simulink model "BSCU"  (R2014b)
settings: Solver=ode45  StartTime=0.0  StopTime=10.0  RelTol=1e-3
undefined symbols (not defined in the file): BRAKE_PRESSURE_LO, BRAKE_PRESSURE_MAX, BRAKE_PRESSURE_MED, LO, MANUAL, MAX, MED
settings Model: CovSFcnEnable=on  Creator=hamza  LastModifiedBy=hbourbou
settings DataIOCC: LimitDataPoints=off  SaveFormat=StructureWithTime
settings DebuggingCC: SolverPrmCheckMsg=none  FrameProcessingCompatibilityMsg=error
settings HardwareCC: ProdBitPerPointer=64  ProdLargestAtomicFloat=Float  ProdIntDivRoundTo=Zero  ProdEndianess=LittleEndian  ProdHWDeviceType=Specified
settings ModelReferenceCC: PropagateSignalLabelsOutOfModel=on

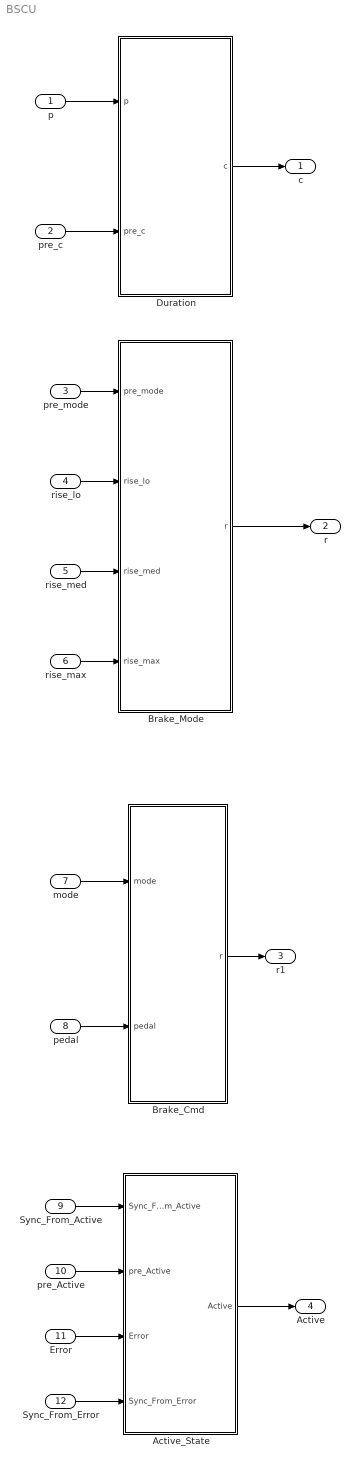
== system BSCU ==
  p : Inport
  pre_c : Inport  Port=2
  pre_mode : Inport  Port=3
  rise_lo : Inport  Port=4
  rise_med : Inport  Port=5
  rise_max : Inport  Port=6
  mode : Inport  Port=7
  pedal : Inport  Port=8
  Sync_From_Active : Inport  Port=9
  pre_Active : Inport  Port=10
  Error : Inport  Port=11
  Sync_From_Error : Inport  Port=12
  Active_State : Stateflow chart  TreatAsAtomicUnit=on
      settings: PermitHierarchicalResolution=ParametersOnly
  Brake_Cmd : Stateflow chart  TreatAsAtomicUnit=on
      settings: PermitHierarchicalResolution=ParametersOnly
  Brake_Mode : Stateflow chart  TreatAsAtomicUnit=on
      settings: PermitHierarchicalResolution=ParametersOnly
  Duration : Stateflow chart  TreatAsAtomicUnit=on
      settings: PermitHierarchicalResolution=ParametersOnly
  c : Outport
  r : Outport  Port=2
  r1 : Outport  Port=3
  Active : Outport  Port=4
  wires:
  p/1 -> Duration/1(p)
  pre_c/1 -> Duration/2(pre_c)
  Duration/1(c) -> c/1
  pre_mode/1 -> Brake_Mode/1(pre_mode)
  rise_lo/1 -> Brake_Mode/2(rise_lo)
  rise_med/1 -> Brake_Mode/3(rise_med)
  rise_max/1 -> Brake_Mode/4(rise_max)
  Brake_Mode/1(r) -> r/1
  mode/1 -> Brake_Cmd/1(mode)
  pedal/1 -> Brake_Cmd/2(pedal)
  Brake_Cmd/1(r) -> r1/1
  Sync_From_Active/1 -> Active_State/1(Sync_From_Active)
  pre_Active/1 -> Active_State/2(pre_Active)
  Error/1 -> Active_State/3(Error)
  Sync_From_Error/1 -> Active_State/4(Sync_From_Error)
  Active_State/1(Active) -> Active/1

== stateflow chart BSCU/Brake_Cmd ==
  (default) -> (junction 4789)
  (junction 4789) -> (junction 4790) [order 1] : [mode == LO]
  (junction 4789) -> (junction 4791) [order 2]
  (junction 4790) -> (junction 4798) : {
      | r = BRAKE_PRESSURE_LO;
      | }
  (junction 4791) -> (junction 4792) [order 1] : [mode == MED ]
  (junction 4791) -> (junction 4793) [order 2]
  (junction 4792) -> (junction 4797) : {
      | r = BRAKE_PRESSURE_MED;
      | }
  (junction 4793) -> (junction 4794) [order 1] : [mode == MAX]
  (junction 4793) -> (junction 4800) [order 2]
  (junction 4794) -> (junction 4796) : {
      | r = BRAKE_PRESSURE_MAX;
      | }
  (junction 4800) -> (junction 4795) : {
      | r = pedal;
      | }
  (junction 4796) -> (junction 4795)
  (junction 4797) -> (junction 4796)
  (junction 4798) -> (junction 4797)
  (junction 4795) -> (junction 4799)
  data: mode input int32; pedal input int32; r output int32; MANUAL parameter =1; LO parameter =2; MED parameter =3; MAX parameter =4; BRAKE_PRESSURE_LO parameter; BRAKE_PRESSURE_MAX parameter; BRAKE_PRESSURE_MED parameter

== stateflow chart BSCU/Brake_Mode ==
  (default) -> (junction 4789)
  (junction 4789) -> (junction 4790) [order 1] : [  ((pre_mode == LO) && rise_lo) || ...
      |    ((pre_mode == MED) && rise_med) || ...
      |    ((pre_mode == MAX) && rise_max)
      | ]
  (junction 4789) -> (junction 4791) [order 2]
  (junction 4790) -> (junction 4798) : {
      | r = MANUAL;
      | }
  (junction 4791) -> (junction 4792) [order 1] : [  (pre_mode != LO) && rise_lo ]
  (junction 4791) -> (junction 4793) [order 2]
  (junction 4792) -> (junction 4797) : {
      | r = LO;
      | }
  (junction 4793) -> (junction 4794) [order 1] : [ (pre_mode != MED) && rise_med ]
  (junction 4793) -> (junction 4800) [order 2]
  (junction 4794) -> (junction 4796) : {
      | r = MED;
      | }
  (junction 4800) -> (junction 4808) [order 1] : [ (pre_mode != MAX) && rise_max ]
  (junction 4800) -> (junction 4795) [order 2] : {
      | r = pre_mode;
      | }
  (junction 4808) -> (junction 4810) : {
      | r = MAX;
      | }
  (junction 4810) -> (junction 4795)
  (junction 4796) -> (junction 4810)
  (junction 4797) -> (junction 4796)
  (junction 4798) -> (junction 4797)
  (junction 4795) -> (junction 4799)
  data: pre_mode input int32; rise_lo input boolean; rise_med input boolean; rise_max input boolean; r output int32; MANUAL parameter =1; LO parameter =2; MED parameter =3; MAX parameter =4

== stateflow chart BSCU/Duration ==
  (default) -> (junction 4827)
  (junction 4827) -> (junction 4828) [order 1] : [p]
  (junction 4827) -> (junction 4829) [order 2] : {c = 0;}
  (junction 4828) -> (junction 4830) : {c = pre_c+1;}
  (junction 4830) -> (junction 4829)
  (junction 4829) -> (junction 4831)
  data: p input boolean; c output int32; pre_c input int32

== stateflow chart BSCU/Active_State ==
  (default) -> (junction 4848)
  (junction 4848) -> (junction 4849) [order 1] : [Error]
  (junction 4848) -> (junction 4850) [order 2]
  (junction 4849) -> (junction 4857) : {Active = false;}
  (junction 4850) -> (junction 4851) [order 1] : [pre_Active && Sync_From_Active && (! Sync_From_Error) && (! Primary_Side) ]
  (junction 4850) -> (junction 4852) [order 2]
  (junction 4851) -> (junction 4856) : {Active = false;}
  (junction 4852) -> (junction 4853) [order 1] : [(!pre_Active) && ( (!Sync_From_Active) || Sync_From_Error)]
  (junction 4852) -> (junction 4854) [order 2] : {Active = pre_Active;}
  (junction 4853) -> (junction 4855) : {Active = true;}
  (junction 4855) -> (junction 4854)
  (junction 4856) -> (junction 4855)
  (junction 4857) -> (junction 4856)
  (junction 4854) -> (junction 4858)
  data: Sync_From_Active input boolean; Active output boolean; pre_Active input boolean; Error input boolean; Sync_From_Error input boolean; Primary_Side parameter
